simulink model "MIR_AUVSimulator_R2021b"  (R2022b)
settings: Solver=ode4  StartTime=SimuParameters.beginning_time_s  StopTime=SimuParameters.simulation_time_s  FixedStep=SimuParameters.sample_time_s  RelTol=1e-3
values from neighbouring files (symbols this model uses):
  command_parameters = loadjson('PilotParameters.json')    [Example_RunSimulation.m]    (also in RunSimulation.m)
  noise = ApplyNoise(SimuParameters.sample_time_s)    [Example_RunSimulation.m]    (also in RunSimulation.m)
  veh_model = loadjson('Conf/AUVParameters.json')    [Example_RunSimulation.m]    (also in RunSimulation.m)
undefined symbols (not defined in the file or in its folder): initial_actuators, initial_state, SimuParameters
libraries: simulink x17
settings Model: PacingRate=10  Creator=seaadh  LastModifiedBy=olanr
settings SolverCC: AlgebraicLoopSolver=TrustRegion
settings DataIOCC: ReturnWorkspaceOutputs=off
settings DebuggingCC: UnconnectedInputMsg=warning  UnconnectedOutputMsg=warning  UnconnectedLineMsg=warning  SFMachineParentedDataDiag=warning  ArithmeticOperatorsInVariantConditions=warning
settings ModelReferenceCC: UpdateModelReferenceTargets=IfOutOfDate  EnableRefExpFcnMdlSchedulingChecks=on  ModelReferenceMinAlgLoopOccurrences=on
settings SFSimCC: SimUseLocalCustomCode=off  CustomCodeUndefinedFunction=UseInterfaceOnly
settings RTWCC: RTWUseLocalCustomCode=off  DLArmComputeVersion=19.05

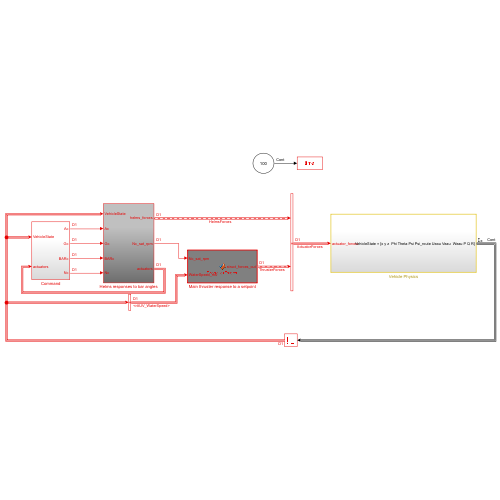
[thumbnail: Simulink's stored preview of the top-level diagram]
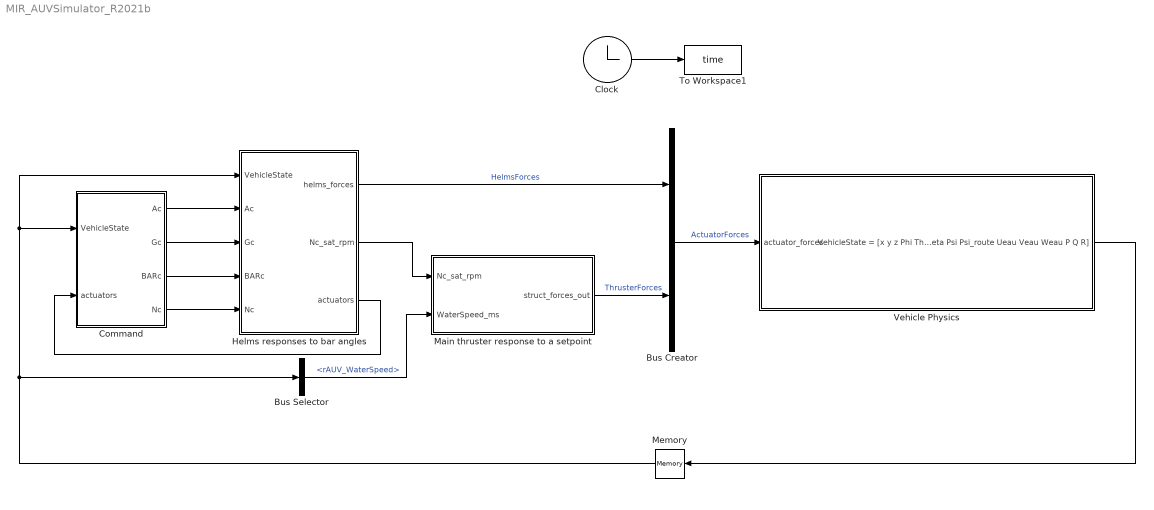
== system MIR_AUVSimulator_R2021b ==
  Bus Creator : BusCreator  Inputs=2  OutDataTypeStr=Bus: ActuatorForces
  Bus Selector : BusSelector  OutputSignals=nu.rAUV_WaterSpeed
  Clock : Clock
  Command : Subsystem
  Helms responses to bar angles : Subsystem
  Main thruster response to a setpoint : MATLAB Function  TreatAsAtomicUnit=on
  Memory : Memory  InitialCondition=initial_state  InheritSampleTime=on
  To Workspace1 : ToWorkspace  VariableName=time  SampleTime=SimuParameters.sample_time_s
  Vehicle Physics : Subsystem  TreatAsAtomicUnit=on
      settings: MinAlgLoopOccurrences=on
  wires:
  Clock/1 -> To Workspace1/1
  Memory/1 -> Helms responses to bar angles/1(VehicleState), Command/1(VehicleState), Bus Selector/1
  Helms responses to bar angles/1(helms_forces) -> Bus Creator/1  "HelmsForces"
  Helms responses to bar angles/2(Nc_sat_rpm) -> Main thruster response to a setpoint/1(Nc_sat_rpm)
  Command/1(Ac) -> Helms responses to bar angles/2(Ac)
  Command/4(Nc) -> Helms responses to bar angles/5(Nc)
  Main thruster response to a setpoint/1(struct_forces_out) -> Bus Creator/2  "ThrusterForces"
  Command/2(Gc) -> Helms responses to bar angles/3(Gc)
  Command/3(BARc) -> Helms responses to bar angles/4(BARc)
  Bus Creator/1 -> Vehicle Physics/1(actuator_forces)  "ActuatorForces"
  Vehicle Physics/1(VehicleState = [x y z Phi Theta Psi Psi_route Ueau Veau Weau P Q R]) -> Memory/1
  Bus Selector/1 -> Main thruster response to a setpoint/2(WaterSpeed_ms)  "<rAUV_WaterSpeed>"
  Helms responses to bar angles/3(actuators) -> Command/2(actuators)

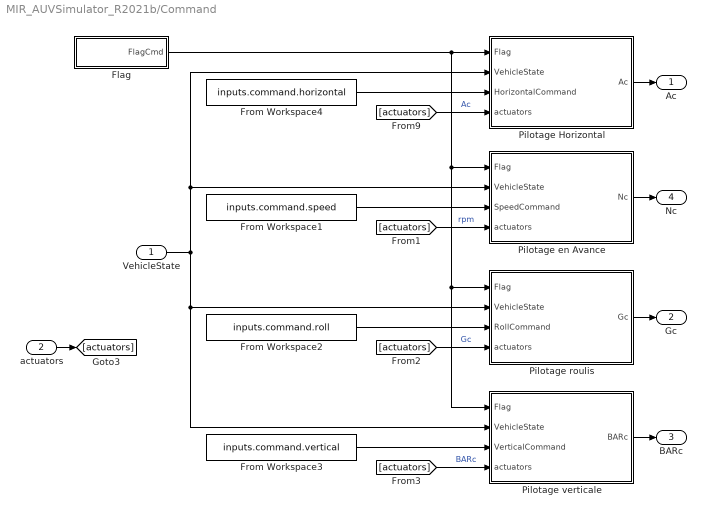
== system MIR_AUVSimulator_R2021b/Command ==
  VehicleState : Inport
  actuators : Inport  Port=2
  Flag : Subsystem
  From Workspace1 : FromWorkspace  VariableName=inputs.command.speed  SampleTime=SimuParameters.sample_time_s  Interpolate=off  OutputAfterFinalValue=Setting to zero
  From Workspace2 : FromWorkspace  VariableName=inputs.command.roll  SampleTime=SimuParameters.sample_time_s  Interpolate=off  OutputAfterFinalValue=Setting to zero
  From Workspace3 : FromWorkspace  VariableName=inputs.command.vertical  SampleTime=SimuParameters.sample_time_s  Interpolate=off  OutputAfterFinalValue=Setting to zero
  From Workspace4 : FromWorkspace  VariableName=inputs.command.horizontal  SampleTime=SimuParameters.sample_time_s  Interpolate=off  OutputAfterFinalValue=Setting to zero
  Pilotage Horizontal : Subsystem  TreatAsAtomicUnit=on  SystemSampleTime=SimuParameters.sample_time_s
  Pilotage en Avance : Subsystem  TreatAsAtomicUnit=on  SystemSampleTime=SimuParameters.sample_time_s
  Pilotage roulis : Subsystem  TreatAsAtomicUnit=on  SystemSampleTime=SimuParameters.sample_time_s
  Pilotage verticale : Subsystem  TreatAsAtomicUnit=on  SystemSampleTime=SimuParameters.sample_time_s
  Ac : Outport  VectorParamsAs1DForOutWhenUnconnected=off
  Gc : Outport  Port=2  VectorParamsAs1DForOutWhenUnconnected=off
  BARc : Outport  Port=3  VectorParamsAs1DForOutWhenUnconnected=off
  Nc : Outport  Port=4  VectorParamsAs1DForOutWhenUnconnected=off
  wires:
  Flag/1(FlagCmd) -> Pilotage verticale/1(Flag), Pilotage roulis/1(Flag), Pilotage en Avance/1(Flag), Pilotage Horizontal/1(Flag)
  Pilotage verticale/1(BARc) -> BARc/1
  Pilotage roulis/1(Gc) -> Gc/1
  Pilotage Horizontal/1(Ac) -> Ac/1
  From Workspace4/1 -> Pilotage Horizontal/3(HorizontalCommand)
  From Workspace3/1 -> Pilotage verticale/3(VerticalCommand)
  Pilotage en Avance/1(Nc) -> Nc/1
  VehicleState/1 -> Pilotage Horizontal/2(VehicleState), Pilotage en Avance/2(VehicleState), Pilotage verticale/2(VehicleState), Pilotage roulis/2(VehicleState)
  From Workspace1/1 -> Pilotage en Avance/3(SpeedCommand)
  From Workspace2/1 -> Pilotage roulis/3(RollCommand)
  actuators/1 -> [actuators]
  [actuators] -> Pilotage Horizontal/4(actuators)  "Ac"
  [actuators] -> Pilotage en Avance/4(actuators)  "rpm"
  [actuators] -> Pilotage roulis/4(actuators)  "Gc"
  [actuators] -> Pilotage verticale/4(actuators)  "BARc"

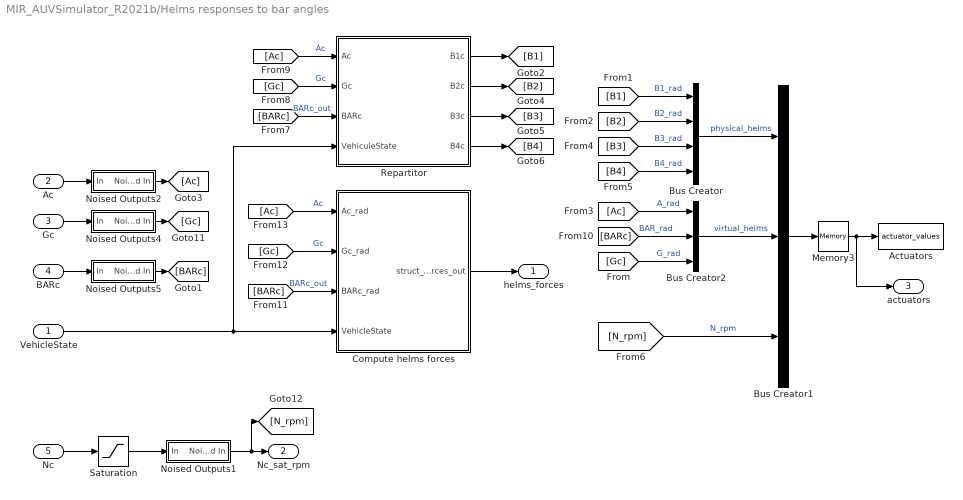
== system MIR_AUVSimulator_R2021b/Helms responses to bar angles ==
  VehicleState : Inport
  Ac : Inport  Port=2
  Gc : Inport  Port=3
  BARc : Inport  Port=4
  Nc : Inport  Port=5
  Actuators : ToWorkspace  VariableName=actuator_values  SaveFormat=Timeseries  SampleTime=SimuParameters.sample_time_s
  Bus Creator : BusCreator  Inputs=4  OutDataTypeStr=Bus: physical_helms
  Bus Creator1 : BusCreator  Inputs=3  OutDataTypeStr=Bus: ActuatorState
  Bus Creator2 : BusCreator  Inputs=3  OutDataTypeStr=Bus: virtual_helms
  Compute helms forces : MATLAB Function  TreatAsAtomicUnit=on
  Memory3 : Memory  InitialCondition=initial_actuators  InheritSampleTime=on
  Noised Outputs1 : Subsystem  mask{noise_variable=noise.RPM}
      mask prompts: noise_variable "Variable to noise"
  Noised Outputs2 : Subsystem  mask{noise_variable=noise.A_rad}
      mask prompts: noise_variable "Variable to noise"
  Noised Outputs4 : Subsystem  mask{noise_variable=noise.G_rad}
      mask prompts: noise_variable "Variable to noise"
  Noised Outputs5 : Subsystem  mask{noise_variable=noise.BAR_rad}
      mask prompts: noise_variable "Variable to noise"
  Repartitor : MATLAB Function  TreatAsAtomicUnit=on  SystemSampleTime=SimuParameters.sample_time_s
  Saturation : Saturate  UpperLimit=veh_model.Propeller.rpm_sat(2)  LowerLimit=veh_model.Propeller.rpm_sat(1)
  helms_forces : Outport  VectorParamsAs1DForOutWhenUnconnected=off
  Nc_sat_rpm : Outport  Port=2  VectorParamsAs1DForOutWhenUnconnected=off
  actuators : Outport  Port=3  VectorParamsAs1DForOutWhenUnconnected=off
  wires:
  VehicleState/1 -> Compute helms forces/4(VehicleState), Repartitor/4(VehiculeState)
  Compute helms forces/1(struct_forces_out) -> helms_forces/1
  Bus Creator1/1 -> Memory3/1
  [B3] -> Bus Creator/3  "B3_rad"
  [B2] -> Bus Creator/2  "B2_rad"
  [B4] -> Bus Creator/4  "B4_rad"
  [B1] -> Bus Creator/1  "B1_rad"
  Saturation/1 -> Noised Outputs1/1(In)
  Noised Outputs1/1(Noised In) -> [N_rpm], Nc_sat_rpm/1
  Repartitor/2(B2c) -> [B2]
  Repartitor/1(B1c) -> [B1]
  Repartitor/3(B3c) -> [B3]
  Repartitor/4(B4c) -> [B4]
  [Ac] -> Compute helms forces/1(Ac_rad)  "Ac"
  [Gc] -> Compute helms forces/2(Gc_rad)  "Gc"
  [Ac] -> Repartitor/1(Ac)  "Ac"
  [Gc] -> Repartitor/2(Gc)  "Gc"
  [BARc] -> Repartitor/3(BARc)  "BARc_out"
  [Ac] -> Bus Creator2/1  "A_rad"
  [BARc] -> Bus Creator2/2  "BAR_rad"
  [Gc] -> Bus Creator2/3  "G_rad"
  [N_rpm] -> Bus Creator1/3  "N_rpm"
  [BARc] -> Compute helms forces/3(BARc_rad)  "BARc_out"
  Bus Creator/1 -> Bus Creator1/1  "physical_helms"
  Bus Creator2/1 -> Bus Creator1/2  "virtual_helms"
  Noised Outputs2/1(Noised In) -> [Ac]
  Noised Outputs4/1(Noised In) -> [Gc]
  Noised Outputs5/1(Noised In) -> [BARc]
  Nc/1 -> Saturation/1
  Ac/1 -> Noised Outputs2/1(In)
  Gc/1 -> Noised Outputs4/1(In)
  BARc/1 -> Noised Outputs5/1(In)
  Memory3/1 -> actuators/1, Actuators/1

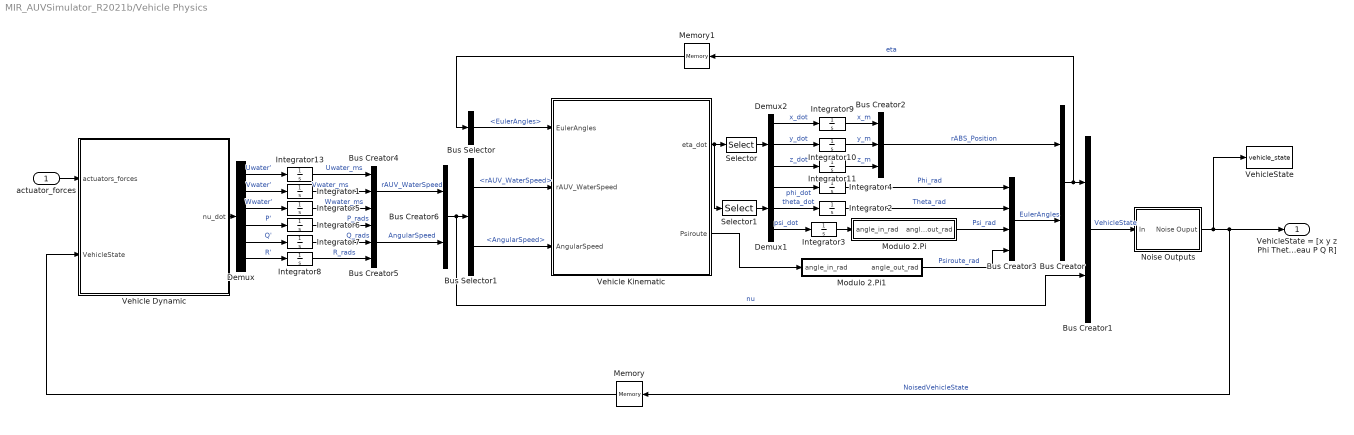
== system MIR_AUVSimulator_R2021b/Vehicle Physics ==
  actuator_forces : Inport
  Bus Creator : BusCreator  Inputs=2  OutDataTypeStr=Bus: eta
  Bus Creator1 : BusCreator  Inputs=2  OutDataTypeStr=Bus: VehicleState
  Bus Creator2 : BusCreator  Inputs=3
  Bus Creator3 : BusCreator  Inputs=4
  Bus Creator4 : BusCreator  Inputs=3
  Bus Creator5 : BusCreator  Inputs=3
  Bus Creator6 : BusCreator  Inputs=2  OutDataTypeStr=Bus: nu
  Bus Selector : BusSelector  OutputSignals=EulerAngles
  Bus Selector1 : BusSelector  OutputSignals=rAUV_WaterSpeed,AngularSpeed
  Demux : Demux  Outputs=6
  Demux1 : Demux  Outputs=3
  Demux2 : Demux  Outputs=3
  Integrator1 : Integrator  InitialCondition=initial_state.nu.rAUV_WaterSpeed.Vwater_ms  ContinuousStateAttributes='Vwater_ms'
  Integrator10 : Integrator  InitialCondition=initial_state.eta.rABS_Position.y_m  ContinuousStateAttributes='y_m'
  Integrator11 : Integrator  InitialCondition=initial_state.eta.rABS_Position.z_m  ContinuousStateAttributes='z_m'
  Integrator13 : Integrator  InitialCondition=initial_state.nu.rAUV_WaterSpeed.Uwater_ms  ContinuousStateAttributes='Uwater_ms'
  Integrator2 : Integrator  InitialCondition=initial_state.eta.EulerAngles.Theta_rad  ContinuousStateAttributes='theta_rad'
  Integrator3 : Integrator  InitialCondition=initial_state.eta.EulerAngles.Psi_rad  ContinuousStateAttributes='psi_rad'
  Integrator4 : Integrator  InitialCondition=initial_state.eta.EulerAngles.Phi_rad  ContinuousStateAttributes='phi_rad'
  Integrator5 : Integrator  InitialCondition=initial_state.nu.rAUV_WaterSpeed.Wwater_ms  ContinuousStateAttributes='Wwater_ms'
  Integrator6 : Integrator  InitialCondition=initial_state.nu.AngularSpeed.P_rads  ContinuousStateAttributes='P_rads'
  Integrator7 : Integrator  InitialCondition=initial_state.nu.AngularSpeed.Q_rads  ContinuousStateAttributes='Q_rads'
  Integrator8 : Integrator  InitialCondition=initial_state.nu.AngularSpeed.R_rads  ContinuousStateAttributes='R_rads'
  Integrator9 : Integrator  InitialCondition=initial_state.eta.rABS_Position.x_m  ContinuousStateAttributes='x_m'
  Memory : Memory  InitialCondition=initial_state  InheritSampleTime=on
  Memory1 : Memory  InitialCondition=initial_state.eta  InheritSampleTime=on
  Modulo 2.Pi : MATLAB Function  TreatAsAtomicUnit=on
  Modulo 2.Pi1 : MATLAB Function  TreatAsAtomicUnit=on
  Noise Outputs : Subsystem
  Selector : Selector  InputPortWidth=6  IndexOptions=Index vector (dialog)  Indices=[1 2 3]  OutputSizes=1
  Selector1 : Selector  InputPortWidth=6  IndexOptions=Index vector (dialog)  Indices=[4 5 6]  OutputSizes=1
  Vehicle Dynamic : Subsystem  TreatAsAtomicUnit=on
  Vehicle Kinematic : MATLAB Function  TreatAsAtomicUnit=on
  VehicleState : ToWorkspace  VariableName=vehicle_state  SaveFormat=Timeseries  SampleTime=SimuParameters.sample_time_s
  VehicleState = [x y z Phi Theta Psi Psi_route Ueau Veau Weau P Q R] : Outport  VectorParamsAs1DForOutWhenUnconnected=off
  wires:
  Demux2/1 -> Integrator9/1  "x_dot"
  Bus Creator4/1 -> Bus Creator6/1  "rAUV_WaterSpeed"
  Demux2/3 -> Integrator11/1  "z_dot"
  Bus Creator5/1 -> Bus Creator6/2  "AngularSpeed"
  Demux/6 -> Integrator8/1  "R'"
  Bus Creator6/1 -> Bus Creator1/2, Bus Selector1/1  "nu"
  Bus Selector1/1 -> Vehicle Kinematic/2(rAUV_WaterSpeed)  "<rAUV_WaterSpeed>"
  Demux/5 -> Integrator7/1  "Q'"
  Demux/2 -> Integrator1/1  "Vwater'"
  Demux/1 -> Integrator13/1  "Uwater'"
  Integrator1/1 -> Bus Creator4/2  "Vwater_ms"
  Demux/4 -> Integrator6/1  "P'"
  Bus Selector1/2 -> Vehicle Kinematic/3(AngularSpeed)  "<AngularSpeed>"
  Bus Creator2/1 -> Bus Creator/1  "rABS_Position"
  Demux2/2 -> Integrator10/1  "y_dot"
  Bus Creator/1 -> Memory1/1, Bus Creator1/1  "eta"
  Integrator5/1 -> Bus Creator4/3  "Wwater_ms"
  Bus Selector/1 -> Vehicle Kinematic/1(EulerAngles)  "<EulerAngles>"
  Bus Creator3/1 -> Bus Creator/2  "EulerAngles"
  Vehicle Dynamic/1(nu_dot) -> Demux/1
  Demux/3 -> Integrator5/1  "Wwater'"
  Bus Creator1/1 -> Noise Outputs/1(In)  "VehicleState"
  Memory/1 -> Vehicle Dynamic/2(VehicleState)
  Integrator8/1 -> Bus Creator5/3  "R_rads"
  Integrator13/1 -> Bus Creator4/1  "Uwater_ms"
  Noise Outputs/1(Noise Ouput) -> VehicleState = [x y z Phi Theta Psi Psi_route Ueau Veau Weau P Q R]/1, Memory/1, VehicleState/1  "NoisedVehicleState"
  Integrator6/1 -> Bus Creator5/1  "P_rads"
  Integrator7/1 -> Bus Creator5/2  "Q_rads"
  Memory1/1 -> Bus Selector/1
  Vehicle Kinematic/1(eta_dot) -> Selector1/1, Selector/1
  actuator_forces/1 -> Vehicle Dynamic/1(actuators_forces)
  Integrator9/1 -> Bus Creator2/1  "x_m"
  Integrator10/1 -> Bus Creator2/2  "y_m"
  Integrator11/1 -> Bus Creator2/3  "z_m"
  Selector/1 -> Demux2/1
  Demux1/3 -> Integrator3/1  "psi_dot"
  Demux1/2 -> Integrator2/1  "theta_dot"
  Demux1/1 -> Integrator4/1  "phi_dot"
  Selector1/1 -> Demux1/1
  Integrator3/1 -> Modulo 2.Pi/1(angle_in_rad)
  Modulo 2.Pi/1(angle_out_rad) -> Bus Creator3/3  "Psi_rad"
  Modulo 2.Pi1/1(angle_out_rad) -> Bus Creator3/4  "Psiroute_rad"
  Vehicle Kinematic/2(Psiroute) -> Modulo 2.Pi1/1(angle_in_rad)
  Integrator4/1 -> Bus Creator3/1  "Phi_rad"
  Integrator2/1 -> Bus Creator3/2  "Theta_rad"

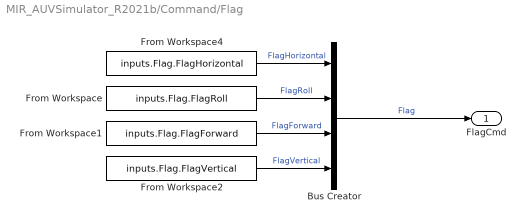
== system MIR_AUVSimulator_R2021b/Command/Flag ==
  Bus Creator : BusCreator  Inputs=4  OutDataTypeStr=Bus: Flag
  From Workspace : FromWorkspace  VariableName=inputs.Flag.FlagRoll  SampleTime=SimuParameters.sample_time_s
  From Workspace1 : FromWorkspace  VariableName=inputs.Flag.FlagForward  SampleTime=SimuParameters.sample_time_s
  From Workspace2 : FromWorkspace  VariableName=inputs.Flag.FlagVertical  SampleTime=SimuParameters.sample_time_s
  From Workspace4 : FromWorkspace  VariableName=inputs.Flag.FlagHorizontal  SampleTime=SimuParameters.sample_time_s
  FlagCmd : Outport  VectorParamsAs1DForOutWhenUnconnected=off
  wires:
  Bus Creator/1 -> FlagCmd/1  "Flag"
  From Workspace4/1 -> Bus Creator/1  "FlagHorizontal"
  From Workspace/1 -> Bus Creator/2  "FlagRoll"
  From Workspace1/1 -> Bus Creator/3  "FlagForward"
  From Workspace2/1 -> Bus Creator/4  "FlagVertical"

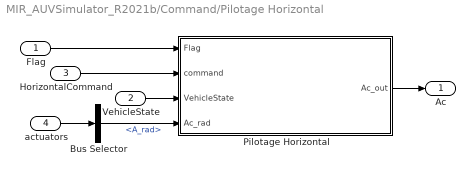
== system MIR_AUVSimulator_R2021b/Command/Pilotage Horizontal ==
  Flag : Inport
  VehicleState : Inport  Port=2
  HorizontalCommand : Inport  Port=3
  actuators : Inport  Port=4
  Bus Selector : BusSelector  OutputSignals=virtual_helms.A_rad
  Pilotage Horizontal : MATLAB Function  TreatAsAtomicUnit=on  SystemSampleTime=SimuParameters.sample_time_s
  Ac : Outport  VectorParamsAs1DForOutWhenUnconnected=off
  wires:
  Pilotage Horizontal/1(Ac_out) -> Ac/1
  HorizontalCommand/1 -> Pilotage Horizontal/2(command)
  VehicleState/1 -> Pilotage Horizontal/3(VehicleState)
  Flag/1 -> Pilotage Horizontal/1(Flag)
  actuators/1 -> Bus Selector/1
  Bus Selector/1 -> Pilotage Horizontal/4(Ac_rad)  "<A_rad>"

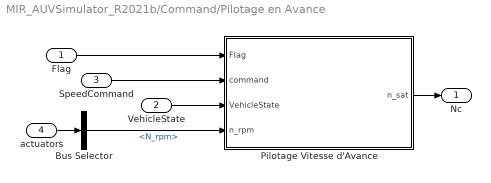
== system MIR_AUVSimulator_R2021b/Command/Pilotage en Avance ==
  Flag : Inport
  VehicleState : Inport  Port=2
  SpeedCommand : Inport  Port=3
  actuators : Inport  Port=4
  Bus Selector : BusSelector  OutputSignals=N_rpm
  Pilotage Vitesse d'Avance : MATLAB Function  TreatAsAtomicUnit=on  SystemSampleTime=SimuParameters.sample_time_s
  Nc : Outport  VectorParamsAs1DForOutWhenUnconnected=off
  wires:
  Pilotage Vitesse d'Avance/1(n_sat) -> Nc/1
  VehicleState/1 -> Pilotage Vitesse d'Avance/3(VehicleState)
  Flag/1 -> Pilotage Vitesse d'Avance/1(Flag)
  SpeedCommand/1 -> Pilotage Vitesse d'Avance/2(command)
  actuators/1 -> Bus Selector/1
  Bus Selector/1 -> Pilotage Vitesse d'Avance/4(n_rpm)  "<N_rpm>"

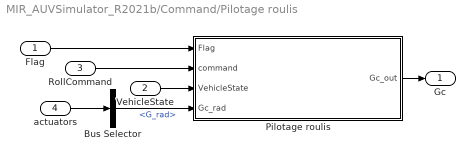
== system MIR_AUVSimulator_R2021b/Command/Pilotage roulis ==
  Flag : Inport
  VehicleState : Inport  Port=2
  RollCommand : Inport  Port=3
  actuators : Inport  Port=4
  Bus Selector : BusSelector  OutputSignals=virtual_helms.G_rad
  Pilotage roulis : MATLAB Function  TreatAsAtomicUnit=on  SystemSampleTime=SimuParameters.sample_time_s
  Gc : Outport  VectorParamsAs1DForOutWhenUnconnected=off
  wires:
  Pilotage roulis/1(Gc_out) -> Gc/1
  Flag/1 -> Pilotage roulis/1(Flag)
  VehicleState/1 -> Pilotage roulis/3(VehicleState)
  RollCommand/1 -> Pilotage roulis/2(command)
  actuators/1 -> Bus Selector/1
  Bus Selector/1 -> Pilotage roulis/4(Gc_rad)  "<G_rad>"

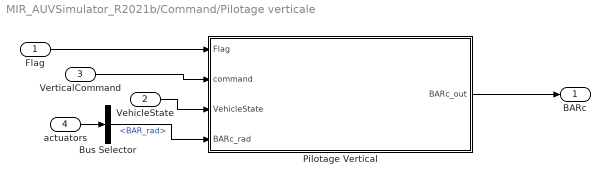
== system MIR_AUVSimulator_R2021b/Command/Pilotage verticale ==
  Flag : Inport
  VehicleState : Inport  Port=2
  VerticalCommand : Inport  Port=3
  actuators : Inport  Port=4
  Bus Selector : BusSelector  OutputSignals=virtual_helms.BAR_rad
  Pilotage Vertical : MATLAB Function  TreatAsAtomicUnit=on  SystemSampleTime=SimuParameters.sample_time_s
  BARc : Outport  VectorParamsAs1DForOutWhenUnconnected=off
  wires:
  Pilotage Vertical/1(BARc_out) -> BARc/1
  Flag/1 -> Pilotage Vertical/1(Flag)
  VehicleState/1 -> Pilotage Vertical/3(VehicleState)
  VerticalCommand/1 -> Pilotage Vertical/2(command)
  actuators/1 -> Bus Selector/1
  Bus Selector/1 -> Pilotage Vertical/4(BARc_rad)  "<BAR_rad>"

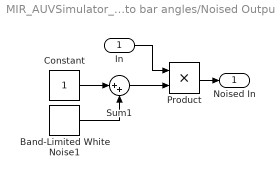
== system MIR_AUVSimulator_R2021b/Helms responses to bar angles/Noised Outputs1 ==
  In : Inport
  Band-Limited White Noise1 : simulink/Sources/Band-Limited White Noise  Cov=noise_variable.noise_power  Ts=SimuParameters.sample_time_s  seed=[23341]
  Constant : Constant
  Product : Product
  Sum1 : Sum  Inputs=|++
  Noised In : Outport  VectorParamsAs1DForOutWhenUnconnected=off
  wires:
  Product/1 -> Noised In/1
  In/1 -> Product/1
  Constant/1 -> Sum1/1
  Band-Limited White Noise1/1 -> Sum1/2
  Sum1/1 -> Product/2

== system MIR_AUVSimulator_R2021b/Helms responses to bar angles/Noised Outputs2 ==
  In : Inport
  Band-Limited White Noise1 : simulink/Sources/Band-Limited White Noise  Cov=noise_variable.noise_power  Ts=SimuParameters.sample_time_s  seed=[23341]
  Constant : Constant
  Product : Product
  Sum1 : Sum  Inputs=|++
  Noised In : Outport  VectorParamsAs1DForOutWhenUnconnected=off
  wires:
  Product/1 -> Noised In/1
  In/1 -> Product/1
  Constant/1 -> Sum1/1
  Band-Limited White Noise1/1 -> Sum1/2
  Sum1/1 -> Product/2

== system MIR_AUVSimulator_R2021b/Helms responses to bar angles/Noised Outputs4 ==
  In : Inport
  Band-Limited White Noise1 : simulink/Sources/Band-Limited White Noise  Cov=noise_variable.noise_power  Ts=SimuParameters.sample_time_s  seed=[23341]
  Constant : Constant
  Product : Product
  Sum1 : Sum  Inputs=|++
  Noised In : Outport  VectorParamsAs1DForOutWhenUnconnected=off
  wires:
  Product/1 -> Noised In/1
  In/1 -> Product/1
  Constant/1 -> Sum1/1
  Band-Limited White Noise1/1 -> Sum1/2
  Sum1/1 -> Product/2

== system MIR_AUVSimulator_R2021b/Helms responses to bar angles/Noised Outputs5 ==
  In : Inport
  Band-Limited White Noise1 : simulink/Sources/Band-Limited White Noise  Cov=noise_variable.noise_power  Ts=SimuParameters.sample_time_s  seed=[23341]
  Constant : Constant
  Product : Product
  Sum1 : Sum  Inputs=|++
  Noised In : Outport  VectorParamsAs1DForOutWhenUnconnected=off
  wires:
  Product/1 -> Noised In/1
  In/1 -> Product/1
  Constant/1 -> Sum1/1
  Band-Limited White Noise1/1 -> Sum1/2
  Sum1/1 -> Product/2

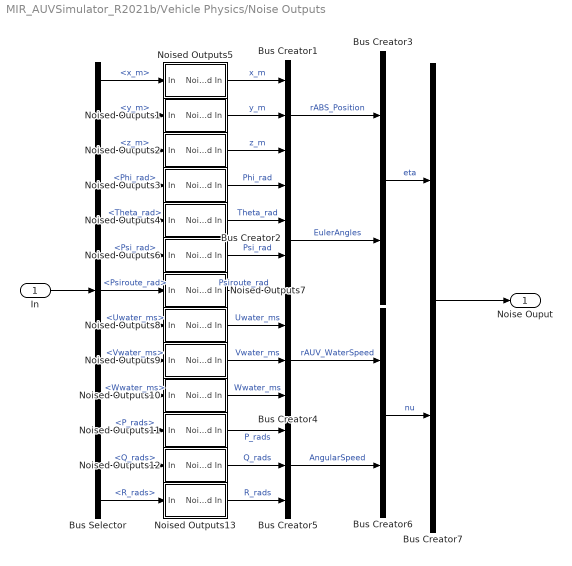
== system MIR_AUVSimulator_R2021b/Vehicle Physics/Noise Outputs ==
  In : Inport
  Bus Creator1 : BusCreator  Inputs=3  OutDataTypeStr=Bus: rABS_Position
  Bus Creator2 : BusCreator  Inputs=4  OutDataTypeStr=Bus: EulerAngles
  Bus Creator3 : BusCreator  Inputs=2  OutDataTypeStr=Bus: eta
  Bus Creator4 : BusCreator  Inputs=3  OutDataTypeStr=Bus: rAUV_WaterSpeed
  Bus Creator5 : BusCreator  Inputs=3  OutDataTypeStr=Bus: AngularSpeed
  Bus Creator6 : BusCreator  Inputs=2  OutDataTypeStr=Bus: nu
  Bus Creator7 : BusCreator  Inputs=2  OutDataTypeStr=Bus: VehicleState
  Bus Selector : BusSelector  OutputSignals=eta.rABS_Position.x_m,eta.rABS_Position.y_m,eta.rABS_Position.z_m,eta.EulerAngles.Phi_rad,eta.EulerAngles.Theta_rad,eta.EulerAngles.Psi_rad,eta.EulerAngles.Psiroute_rad,nu.rAUV_WaterSpeed.Uwater_ms,nu.rAUV_WaterSpeed.Vwater_ms,nu.rAUV_WaterSpeed.Wwater_ms,nu.AngularSpeed.P_rads,nu.AngularSpeed.Q_rads,nu.AngularSpeed.R_rads
  Noised Outputs1 : Subsystem  mask{noise_variable=noise.y_m}
      mask prompts: noise_variable "Variable to noise"
  Noised Outputs10 : Subsystem  mask{noise_variable=noise.Weau_ms}
      mask prompts: noise_variable "Variable to noise"
  Noised Outputs11 : Subsystem  mask{noise_variable=noise.P_rads}
      mask prompts: noise_variable "Variable to noise"
  Noised Outputs12 : Subsystem  mask{noise_variable=noise.Q_rads}
      mask prompts: noise_variable "Variable to noise"
  Noised Outputs13 : Subsystem  mask{noise_variable=noise.R_rads}
      mask prompts: noise_variable "Variable to noise"
  Noised Outputs2 : Subsystem  mask{noise_variable=noise.z_m}
      mask prompts: noise_variable "Variable to noise"
  Noised Outputs3 : Subsystem  mask{noise_variable=noise.Phi_rad}
      mask prompts: noise_variable "Variable to noise"
  Noised Outputs4 : Subsystem  mask{noise_variable=noise.Theta_rad}
      mask prompts: noise_variable "Variable to noise"
  Noised Outputs5 : Subsystem  mask{noise_variable=noise.x_m}
      mask prompts: noise_variable "Variable to noise"
  Noised Outputs6 : Subsystem  mask{noise_variable=noise.Psi_rad}
      mask prompts: noise_variable "Variable to noise"
  Noised Outputs7 : Subsystem  mask{noise_variable=noise.Psiroute_rad}
      mask prompts: noise_variable "Variable to noise"
  Noised Outputs8 : Subsystem  mask{noise_variable=noise.Ueau_ms}
      mask prompts: noise_variable "Variable to noise"
  Noised Outputs9 : Subsystem  mask{noise_variable=noise.Veau_ms}
      mask prompts: noise_variable "Variable to noise"
  Noise Ouput : Outport  VectorParamsAs1DForOutWhenUnconnected=off
  wires:
  Noised Outputs9/1(Noised In) -> Bus Creator4/2  "Vwater_ms"
  Noised Outputs8/1(Noised In) -> Bus Creator4/1  "Uwater_ms"
  Noised Outputs10/1(Noised In) -> Bus Creator4/3  "Wwater_ms"
  Bus Creator5/1 -> Bus Creator6/2  "AngularSpeed"
  Bus Creator4/1 -> Bus Creator6/1  "rAUV_WaterSpeed"
  Noised Outputs11/1(Noised In) -> Bus Creator5/1  "P_rads"
  Noised Outputs12/1(Noised In) -> Bus Creator5/2  "Q_rads"
  Noised Outputs13/1(Noised In) -> Bus Creator5/3  "R_rads"
  Bus Creator3/1 -> Bus Creator7/1  "eta"
  Bus Creator2/1 -> Bus Creator3/2  "EulerAngles"
  Noised Outputs5/1(Noised In) -> Bus Creator1/1  "x_m"
  Bus Creator1/1 -> Bus Creator3/1  "rABS_Position"
  Noised Outputs1/1(Noised In) -> Bus Creator1/2  "y_m"
  Noised Outputs2/1(Noised In) -> Bus Creator1/3  "z_m"
  Noised Outputs3/1(Noised In) -> Bus Creator2/1  "Phi_rad"
  Noised Outputs6/1(Noised In) -> Bus Creator2/3  "Psi_rad"
  Noised Outputs4/1(Noised In) -> Bus Creator2/2  "Theta_rad"
  In/1 -> Bus Selector/1
  Bus Creator7/1 -> Noise Ouput/1
  Bus Selector/1 -> Noised Outputs5/1(In)  "<x_m>"
  Bus Selector/2 -> Noised Outputs1/1(In)  "<y_m>"
  Bus Selector/3 -> Noised Outputs2/1(In)  "<z_m>"
  Bus Selector/4 -> Noised Outputs3/1(In)  "<Phi_rad>"
  Bus Selector/5 -> Noised Outputs4/1(In)  "<Theta_rad>"
  Bus Selector/6 -> Noised Outputs6/1(In)  "<Psi_rad>"
  Bus Selector/7 -> Noised Outputs7/1(In)  "<Psiroute_rad>"
  Noised Outputs7/1(Noised In) -> Bus Creator2/4  "Psiroute_rad"
  Bus Creator6/1 -> Bus Creator7/2  "nu"
  Bus Selector/8 -> Noised Outputs8/1(In)  "<Uwater_ms>"
  Bus Selector/9 -> Noised Outputs9/1(In)  "<Vwater_ms>"
  Bus Selector/10 -> Noised Outputs10/1(In)  "<Wwater_ms>"
  Bus Selector/11 -> Noised Outputs11/1(In)  "<P_rads>"
  Bus Selector/12 -> Noised Outputs12/1(In)  "<Q_rads>"
  Bus Selector/13 -> Noised Outputs13/1(In)  "<R_rads>"

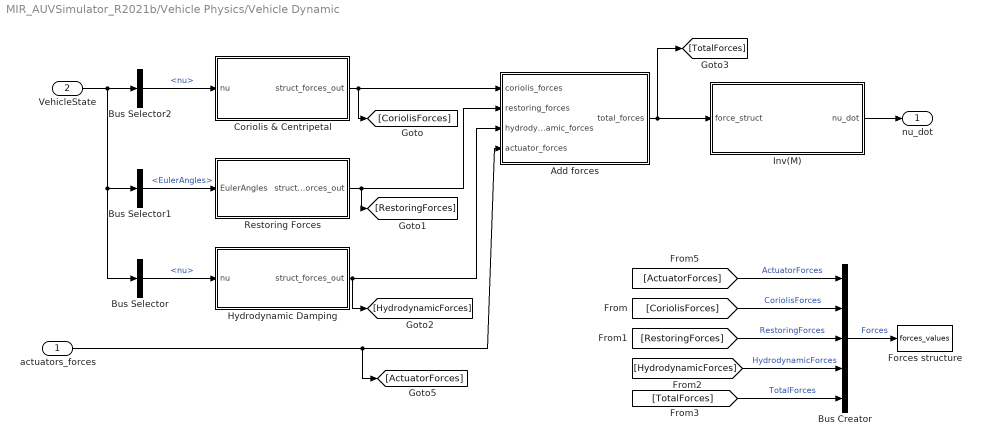
== system MIR_AUVSimulator_R2021b/Vehicle Physics/Vehicle Dynamic ==
  actuators_forces : Inport
  VehicleState : Inport  Port=2
  Add forces : MATLAB Function  TreatAsAtomicUnit=on
  Bus Creator : BusCreator  Inputs=5  OutDataTypeStr=Bus: Forces
  Bus Selector : BusSelector  OutputSignals=nu
  Bus Selector1 : BusSelector  OutputSignals=eta.EulerAngles
  Bus Selector2 : BusSelector  OutputSignals=nu
  Coriolis & Centripetal : MATLAB Function  TreatAsAtomicUnit=on
  Forces structure : ToWorkspace  VariableName=forces_values  SaveFormat=Timeseries  SampleTime=SimuParameters.sample_time_s
  Hydrodynamic Damping : MATLAB Function  TreatAsAtomicUnit=on
  Inv(M) : MATLAB Function  TreatAsAtomicUnit=on
  Restoring Forces : MATLAB Function  TreatAsAtomicUnit=on
  nu_dot : Outport  VectorParamsAs1DForOutWhenUnconnected=off
  wires:
  VehicleState/1 -> Bus Selector2/1, Bus Selector/1, Bus Selector1/1
  Inv(M)/1(nu_dot) -> nu_dot/1
  Bus Selector/1 -> Hydrodynamic Damping/1(nu)  "<nu>"
  Bus Selector2/1 -> Coriolis & Centripetal/1(nu)  "<nu>"
  Bus Selector1/1 -> Restoring Forces/1(EulerAngles)  "<EulerAngles>"
  Coriolis & Centripetal/1(struct_forces_out) -> [CoriolisForces], Add forces/1(coriolis_forces)
  Restoring Forces/1(struct_forces_out) -> Add forces/2(restoring_forces), [RestoringForces]
  Hydrodynamic Damping/1(struct_forces_out) -> [HydrodynamicForces], Add forces/3(hydrodynamic_forces)
  [ActuatorForces] -> Bus Creator/1  "ActuatorForces"
  [CoriolisForces] -> Bus Creator/2  "CoriolisForces"
  [RestoringForces] -> Bus Creator/3  "RestoringForces"
  Bus Creator/1 -> Forces structure/1  "Forces"
  actuators_forces/1 -> Add forces/4(actuator_forces), [ActuatorForces]
  [HydrodynamicForces] -> Bus Creator/4  "HydrodynamicForces"
  [TotalForces] -> Bus Creator/5  "TotalForces"
  Add forces/1(total_forces) -> Inv(M)/1(force_struct), [TotalForces]

== system MIR_AUVSimulator_R2021b/Vehicle Physics/Noise Outputs/Noised Outputs1 ==
  In : Inport
  Band-Limited White Noise1 : simulink/Sources/Band-Limited White Noise  Cov=noise_variable.noise_power  Ts=SimuParameters.sample_time_s  seed=[23341]
  Constant : Constant
  Product : Product
  Sum1 : Sum  Inputs=|++
  Noised In : Outport  VectorParamsAs1DForOutWhenUnconnected=off
  wires:
  Product/1 -> Noised In/1
  In/1 -> Product/1
  Constant/1 -> Sum1/1
  Band-Limited White Noise1/1 -> Sum1/2
  Sum1/1 -> Product/2

== system MIR_AUVSimulator_R2021b/Vehicle Physics/Noise Outputs/Noised Outputs10 ==
  In : Inport
  Band-Limited White Noise1 : simulink/Sources/Band-Limited White Noise  Cov=noise_variable.noise_power  Ts=SimuParameters.sample_time_s  seed=[23341]
  Constant : Constant
  Product : Product
  Sum1 : Sum  Inputs=|++
  Noised In : Outport  VectorParamsAs1DForOutWhenUnconnected=off
  wires:
  Product/1 -> Noised In/1
  In/1 -> Product/1
  Constant/1 -> Sum1/1
  Band-Limited White Noise1/1 -> Sum1/2
  Sum1/1 -> Product/2

== system MIR_AUVSimulator_R2021b/Vehicle Physics/Noise Outputs/Noised Outputs11 ==
  In : Inport
  Band-Limited White Noise1 : simulink/Sources/Band-Limited White Noise  Cov=noise_variable.noise_power  Ts=SimuParameters.sample_time_s  seed=[23341]
  Constant : Constant
  Product : Product
  Sum1 : Sum  Inputs=|++
  Noised In : Outport  VectorParamsAs1DForOutWhenUnconnected=off
  wires:
  Product/1 -> Noised In/1
  In/1 -> Product/1
  Constant/1 -> Sum1/1
  Band-Limited White Noise1/1 -> Sum1/2
  Sum1/1 -> Product/2

== system MIR_AUVSimulator_R2021b/Vehicle Physics/Noise Outputs/Noised Outputs12 ==
  In : Inport
  Band-Limited White Noise1 : simulink/Sources/Band-Limited White Noise  Cov=noise_variable.noise_power  Ts=SimuParameters.sample_time_s  seed=[23341]
  Constant : Constant
  Product : Product
  Sum1 : Sum  Inputs=|++
  Noised In : Outport  VectorParamsAs1DForOutWhenUnconnected=off
  wires:
  Product/1 -> Noised In/1
  In/1 -> Product/1
  Constant/1 -> Sum1/1
  Band-Limited White Noise1/1 -> Sum1/2
  Sum1/1 -> Product/2

== system MIR_AUVSimulator_R2021b/Vehicle Physics/Noise Outputs/Noised Outputs13 ==
  In : Inport
  Band-Limited White Noise1 : simulink/Sources/Band-Limited White Noise  Cov=noise_variable.noise_power  Ts=SimuParameters.sample_time_s  seed=[23341]
  Constant : Constant
  Product : Product
  Sum1 : Sum  Inputs=|++
  Noised In : Outport  VectorParamsAs1DForOutWhenUnconnected=off
  wires:
  Product/1 -> Noised In/1
  In/1 -> Product/1
  Constant/1 -> Sum1/1
  Band-Limited White Noise1/1 -> Sum1/2
  Sum1/1 -> Product/2

== system MIR_AUVSimulator_R2021b/Vehicle Physics/Noise Outputs/Noised Outputs2 ==
  In : Inport
  Band-Limited White Noise1 : simulink/Sources/Band-Limited White Noise  Cov=noise_variable.noise_power  Ts=SimuParameters.sample_time_s  seed=[23341]
  Constant : Constant
  Product : Product
  Sum1 : Sum  Inputs=|++
  Noised In : Outport  VectorParamsAs1DForOutWhenUnconnected=off
  wires:
  Product/1 -> Noised In/1
  In/1 -> Product/1
  Constant/1 -> Sum1/1
  Band-Limited White Noise1/1 -> Sum1/2
  Sum1/1 -> Product/2

== system MIR_AUVSimulator_R2021b/Vehicle Physics/Noise Outputs/Noised Outputs3 ==
  In : Inport
  Band-Limited White Noise1 : simulink/Sources/Band-Limited White Noise  Cov=noise_variable.noise_power  Ts=SimuParameters.sample_time_s  seed=[23341]
  Constant : Constant
  Product : Product
  Sum1 : Sum  Inputs=|++
  Noised In : Outport  VectorParamsAs1DForOutWhenUnconnected=off
  wires:
  Product/1 -> Noised In/1
  In/1 -> Product/1
  Constant/1 -> Sum1/1
  Band-Limited White Noise1/1 -> Sum1/2
  Sum1/1 -> Product/2

== system MIR_AUVSimulator_R2021b/Vehicle Physics/Noise Outputs/Noised Outputs4 ==
  In : Inport
  Band-Limited White Noise1 : simulink/Sources/Band-Limited White Noise  Cov=noise_variable.noise_power  Ts=SimuParameters.sample_time_s  seed=[23341]
  Constant : Constant
  Product : Product
  Sum1 : Sum  Inputs=|++
  Noised In : Outport  VectorParamsAs1DForOutWhenUnconnected=off
  wires:
  Product/1 -> Noised In/1
  In/1 -> Product/1
  Constant/1 -> Sum1/1
  Band-Limited White Noise1/1 -> Sum1/2
  Sum1/1 -> Product/2

== system MIR_AUVSimulator_R2021b/Vehicle Physics/Noise Outputs/Noised Outputs5 ==
  In : Inport
  Band-Limited White Noise1 : simulink/Sources/Band-Limited White Noise  Cov=noise_variable.noise_power  Ts=SimuParameters.sample_time_s  seed=[23341]
  Constant : Constant
  Product : Product
  Sum1 : Sum  Inputs=|++
  Noised In : Outport  VectorParamsAs1DForOutWhenUnconnected=off
  wires:
  Product/1 -> Noised In/1
  In/1 -> Product/1
  Constant/1 -> Sum1/1
  Band-Limited White Noise1/1 -> Sum1/2
  Sum1/1 -> Product/2

== system MIR_AUVSimulator_R2021b/Vehicle Physics/Noise Outputs/Noised Outputs6 ==
  In : Inport
  Band-Limited White Noise1 : simulink/Sources/Band-Limited White Noise  Cov=noise_variable.noise_power  Ts=SimuParameters.sample_time_s  seed=[23341]
  Constant : Constant
  Product : Product
  Sum1 : Sum  Inputs=|++
  Noised In : Outport  VectorParamsAs1DForOutWhenUnconnected=off
  wires:
  Product/1 -> Noised In/1
  In/1 -> Product/1
  Constant/1 -> Sum1/1
  Band-Limited White Noise1/1 -> Sum1/2
  Sum1/1 -> Product/2

== system MIR_AUVSimulator_R2021b/Vehicle Physics/Noise Outputs/Noised Outputs7 ==
  In : Inport
  Band-Limited White Noise1 : simulink/Sources/Band-Limited White Noise  Cov=noise_variable.noise_power  Ts=SimuParameters.sample_time_s  seed=[23341]
  Constant : Constant
  Product : Product
  Sum1 : Sum  Inputs=|++
  Noised In : Outport  VectorParamsAs1DForOutWhenUnconnected=off
  wires:
  Product/1 -> Noised In/1
  In/1 -> Product/1
  Constant/1 -> Sum1/1
  Band-Limited White Noise1/1 -> Sum1/2
  Sum1/1 -> Product/2

== system MIR_AUVSimulator_R2021b/Vehicle Physics/Noise Outputs/Noised Outputs8 ==
  In : Inport
  Band-Limited White Noise1 : simulink/Sources/Band-Limited White Noise  Cov=noise_variable.noise_power  Ts=SimuParameters.sample_time_s  seed=[23341]
  Constant : Constant
  Product : Product
  Sum1 : Sum  Inputs=|++
  Noised In : Outport  VectorParamsAs1DForOutWhenUnconnected=off
  wires:
  Product/1 -> Noised In/1
  In/1 -> Product/1
  Constant/1 -> Sum1/1
  Band-Limited White Noise1/1 -> Sum1/2
  Sum1/1 -> Product/2

== system MIR_AUVSimulator_R2021b/Vehicle Physics/Noise Outputs/Noised Outputs9 ==
  In : Inport
  Band-Limited White Noise1 : simulink/Sources/Band-Limited White Noise  Cov=noise_variable.noise_power  Ts=SimuParameters.sample_time_s  seed=[23341]
  Constant : Constant
  Product : Product
  Sum1 : Sum  Inputs=|++
  Noised In : Outport  VectorParamsAs1DForOutWhenUnconnected=off
  wires:
  Product/1 -> Noised In/1
  In/1 -> Product/1
  Constant/1 -> Sum1/1
  Band-Limited White Noise1/1 -> Sum1/2
  Sum1/1 -> Product/2

== matlab function MIR_AUVSimulator_R2021b/Command/Pilotage en Avance/Pilotage Vitesse d'Avance ==
  data: Flag input; command input; VehicleState input; n_rpm input; n_sat output; SimuParameters parameter; command_parameters parameter
function n_sat = ForwardControl(Flag,command,VehicleState,n_rpm,SimuParameters,command_parameters)

persistent init memory;

speed_flag = GetFlagName(Flag.FlagForward);

%% Load inputs
in.u_ms = VehicleState.nu.rAUV_WaterSpeed.Uwater_ms;
in.uc_ms = command;
in.delta_time_s = SimuParameters.sample_time_s;

%% Memory management
if isempty(init)
    init = false;
    memory = InitPilotForwardSpeed();
end
if init
    init = false;
    memory = InitPilotForwardSpeed();
end

%% Piloting
switch speed_flag
    case 'OpenLoop'
        n_rpm = command;
        init = true;
        
    case 'ForwardSpeed'
        memory = UpdatePilotForwardSpeedMemory(in,memory,command_parameters.ForwardSpeed);
        
        out = PilotForwardSpeed(in,memory,command_parameters.ForwardSpeed);
        n_rpm = out.Nc_rpm;
end

n_sat = n_rpm;
end
function forward_speed_flag = GetFlagName(flag)
% Get the forward_speed_flag string depending on flag numeric input
forward_speed_flag = '';

switch flag
    case 0
        forward_speed_flag = 'OpenLoop';
    case 1
        forward_speed_flag = 'ForwardSpeed';   
end
end

== matlab function MIR_AUVSimulator_R2021b/Helms responses to bar angles/Compute helms forces ==
  data: Ac_rad input; Gc_rad input; BARc_rad input; VehicleState input; struct_forces_out output Bus: HelmsForces; veh_model parameter
function struct_forces_out = HelmsForces(Ac_rad,Gc_rad,BARc_rad,VehicleState,veh_model)
% Be careful. Output need to be a struct (because bus) not an array

u_ms = VehicleState.nu.rAUV_WaterSpeed.Uwater_ms;
v_ms = VehicleState.nu.rAUV_WaterSpeed.Vwater_ms;
w_ms = VehicleState.nu.rAUV_WaterSpeed.Wwater_ms;

speed_ms = [u_ms;v_ms;w_ms]; %m/s
virtual_helms = [Ac_rad;Gc_rad;BARc_rad];

%% Compute the force created by the helms
helm_param = veh_model.XRearHelms;
helm_param.Rho = veh_model.Environment.Rho;
helm_param.Sref = veh_model.Mecanic.surface_reference;
helm_param.Lref = veh_model.Mecanic.length_reference;

helms_forces = ComputeHelmsForce(helm_param, virtual_helms, speed_ms);
            
% Construct the struct output
struct_forces_out.Fx_N = helms_forces(1);
struct_forces_out.Fy_N = helms_forces(2);
struct_forces_out.Fz_N = helms_forces(3);
struct_forces_out.Mx_Nm = helms_forces(4);
struct_forces_out.My_Nm = helms_forces(5);
struct_forces_out.Mz_Nm = helms_forces(6);
end

== matlab function MIR_AUVSimulator_R2021b/Command/Pilotage verticale/Pilotage Vertical ==
  data: Flag input; command input; VehicleState input; BARc_rad input; BARc_out output; command_parameters parameter; SimuParameters parameter; veh_model parameter
function BARc_out  = VerticalControl(Flag,command,VehicleState,BARc_rad,command_parameters,SimuParameters, veh_model)

persistent init memory;

vertical_flag = GetFlagName(Flag.FlagVertical);

%% Load inputs
in.u_ms = VehicleState.nu.rAUV_WaterSpeed.Uwater_ms;
in.w_ms = VehicleState.nu.rAUV_WaterSpeed.Wwater_ms;
in.q_rads = VehicleState.nu.AngularSpeed.Q_rads;
in.theta_rad = VehicleState.eta.EulerAngles.Theta_rad;
in.z_m = VehicleState.eta.rABS_Position.z_m;
in.thetac_rad = 0.0;
in.zc_m = 0.0;
in.delta_time_s = SimuParameters.sample_time_s;

%% Memory management
if isempty(init)
    init = true;
    BARc_rad = 0;
    memory = InitPilotDepth();
end
if init
    init = false;
    memory = InitPilotDepth();
end

%% Piloting
switch vertical_flag
    case 'OpenLoop'
        BARc_rad = command;
        init = true;
        
    case 'Depth'
        in.zc_m = command;
        depth_param = command_parameters.Vertical.Depth;
        
        memory = UpdatePilotDepthMemory(in,memory,depth_param);
        
        out = PilotDepth_LQR(in,memory, depth_param, veh_model);
        BARc_rad = out.BARc;
        
    case 'Pitch'
        in.thetac_rad = command;
        
        out = PilotPitch(in, command_parameters.Vertical.Pitch);
        BARc_rad = out.BARc;
        init = true;
end

BARc_out = BARc_rad;
end


function vertical_flag = GetFlagName(flag)
% Get the vertical_flag string depending on flag numeric input
vertical_flag = '';

switch flag
    case 0
        vertical_flag = 'OpenLoop';
    case 1
        vertical_flag = 'Depth';
    case 2
        vertical_flag = 'Pitch';
end
end

== matlab function MIR_AUVSimulator_R2021b/Vehicle Physics/Vehicle Dynamic/Inv(M) ==
  data: force_struct input; nu_dot output; veh_model parameter
function nu_dot = fcn(force_struct,veh_model)

forces_vector = [...
    force_struct.Fx_N; force_struct.Fy_N; force_struct.Fz_N; ...
    force_struct.Mx_Nm; force_struct.My_Nm; force_struct.Mz_Nm];

inverse_veh_mass_matrix = GetInverseVehicleMassMatrix(veh_model.Mecanic);
nu_dot = inverse_veh_mass_matrix*forces_vector ;
end

== matlab function MIR_AUVSimulator_R2021b/Vehicle Physics/Vehicle Kinematic ==
  data: eta_dot output; EulerAngles input; rAUV_WaterSpeed input; AngularSpeed input; Psiroute output
function [eta_dot, Psiroute] = fcn(EulerAngles,rAUV_WaterSpeed,AngularSpeed)

%% Load inputs and variables
% Remember : EulerAngles = [phi theta psi]' = eta(4:6)
phi_rad = EulerAngles.Phi_rad;
theta_rad = EulerAngles.Theta_rad;
psi_rad = EulerAngles.Psi_rad;

% Remember : nu = [U V W P Q R]' = StateVector(7:12)
waterSpeed_RAUV_ms = [  rAUV_WaterSpeed.Uwater_ms;...
    rAUV_WaterSpeed.Vwater_ms;...
    rAUV_WaterSpeed.Wwater_ms];
angularSpeed_RAUV_rads = [  AngularSpeed.P_rads;...
    AngularSpeed.Q_rads;...
    AngularSpeed.R_rads];

%% Euler angle representation
nu = [waterSpeed_RAUV_ms;angularSpeed_RAUV_rads];

% Calculation of kinematic equations (Fossen 2.38), in radian
J = eulerang(phi_rad,theta_rad,psi_rad);
eta_dot = J*nu;

%% We had the COG (course over ground)
Psiroute = atan2(eta_dot(2),eta_dot(1));
end

== matlab function MIR_AUVSimulator_R2021b/Vehicle Physics/Vehicle Dynamic/Coriolis & Centripetal ==
  data: nu input; struct_forces_out output Bus: CoriolisForces; veh_model parameter

function struct_forces_out = FCoriolis(nu,veh_model)
% Be careful. output need to be a struct (because bus) not an array

%% Get speeds
speed_ms =  [  nu.rAUV_WaterSpeed.Uwater_ms;
    nu.rAUV_WaterSpeed.Vwater_ms;
    nu.rAUV_WaterSpeed.Wwater_ms;];

angular_speed_rads = [nu.AngularSpeed.P_rads;
    nu.AngularSpeed.Q_rads;
    nu.AngularSpeed.R_rads];

%% Compute forces
center_of_gravity_veh_ref = veh_model.Mecanic.center_of_gravity_veh_ref;
mass_kg =  veh_model.Mecanic.mass;
inertia_matrix =  veh_model.Mecanic.inertia_matrix;

coriolis_forces = ComputeCoriolisForces(speed_ms,angular_speed_rads, ...
    center_of_gravity_veh_ref, mass_kg,inertia_matrix);

% Construct the struct output
struct_forces_out.Fx_N = coriolis_forces(1);
struct_forces_out.Fy_N = coriolis_forces(2);
struct_forces_out.Fz_N = coriolis_forces(3);
struct_forces_out.Mx_Nm = coriolis_forces(4);
struct_forces_out.My_Nm = coriolis_forces(5);
struct_forces_out.Mz_Nm = coriolis_forces(6);

end

== matlab function MIR_AUVSimulator_R2021b/Vehicle Physics/Vehicle Dynamic/Hydrodynamic Damping ==
  data: nu input; struct_forces_out output Bus: HydrodynamicForces; veh_model parameter
function struct_forces_out = fcn(nu,veh_model)
% Be careful. output need to be a struct (because bus) not an array

%% Definition of velocity (speed and angular speed) vectors
% Remember nu=[Ueau Veau Weau P Q R]'
Uwater_ms = nu.rAUV_WaterSpeed.Uwater_ms;
Vwater_ms = nu.rAUV_WaterSpeed.Vwater_ms;
Wwater_ms = nu.rAUV_WaterSpeed.Wwater_ms;
P_rads = nu.AngularSpeed.P_rads;
Q_rads = nu.AngularSpeed.Q_rads;
R_rads = nu.AngularSpeed.R_rads;

speed_ms = [Uwater_ms; Vwater_ms; Wwater_ms];
angular_speed_rads = [P_rads; Q_rads; R_rads];

%% Create parameters
parameters = veh_model.Hydrodynamic;
parameters.Lref = veh_model.Mecanic.length_reference;
parameters.Sref = veh_model.Mecanic.surface_reference;
parameters.Rho = veh_model.Environment.Rho;
parameters.nu = veh_model.Environment.nu;

%% Compute Hydrodynamic damping forces
hydrodynamic_forces = ComputeHydrodynamicForce(speed_ms,angular_speed_rads,parameters);

% Construct the struct output
struct_forces_out.Fx_N = hydrodynamic_forces(1);
struct_forces_out.Fy_N = hydrodynamic_forces(2);
struct_forces_out.Fz_N = hydrodynamic_forces(3);
struct_forces_out.Mx_Nm = hydrodynamic_forces(4);
struct_forces_out.My_Nm = hydrodynamic_forces(5);
struct_forces_out.Mz_Nm = hydrodynamic_forces(6);
end

== matlab function MIR_AUVSimulator_R2021b/Vehicle Physics/Vehicle Dynamic/Restoring Forces ==
  data: EulerAngles input; struct_forces_out output Bus: RestoringForces; veh_model parameter
function struct_forces_out  = fcn(EulerAngles,veh_model)
% Be careful. output need to be a struct (because bus) not an array

% Simplified expression of the vector of hydrostatic forces and moments (Fossen 3.120)
restoring_forces = ComputeRestoringForce(EulerAngles,veh_model);

% Construct the struct output
struct_forces_out.Fx_N = restoring_forces(1);
struct_forces_out.Fy_N = restoring_forces(2);
struct_forces_out.Fz_N = restoring_forces(3);
struct_forces_out.Mx_Nm = restoring_forces(4);
struct_forces_out.My_Nm = restoring_forces(5);
struct_forces_out.Mz_Nm = restoring_forces(6);

end

== matlab function MIR_AUVSimulator_R2021b/Command/Pilotage Horizontal/Pilotage Horizontal ==
  data: Flag input; command input; VehicleState input; Ac_rad input; Ac_out output; command_parameters parameter; SimuParameters parameter
function Ac_out = HorizontalControl(Flag,command,VehicleState,Ac_rad,command_parameters,SimuParameters)

persistent init memory;

horizontal_flag = GetFlagName(Flag.FlagHorizontal);

%% Load inputs
in.u_ms = VehicleState.nu.rAUV_WaterSpeed.Uwater_ms;
in.v_ms = VehicleState.nu.rAUV_WaterSpeed.Vwater_ms;
in.r_rads = VehicleState.nu.AngularSpeed.R_rads;
in.psi_rad = VehicleState.eta.EulerAngles.Psi_rad;
in.psic_rad = command;
in.delta_time_s = SimuParameters.sample_time_s;

%% Memory management
if isempty(init)
    init = false;
    memory = InitPilotHeading();
    Ac_rad = 0;
end
if init
    init = false;
    memory = InitPilotHeading();
end

%% Piloting
switch horizontal_flag
    case 'OpenLoop'
        Ac_rad = command;
        init = true;
        
    case 'Heading'
        horizontal_param = command_parameters.Horizontal.Heading;
        memory = UpdatePilotHeadingMemory(in, memory, horizontal_param);
        
        out = PilotHeading(in, memory, horizontal_param);
        Ac_rad = out.Ac;
end
Ac_out = Ac_rad;
end

function horizontal_flag = GetFlagName(flag)
% Get the horizontal_flag string depending on flag numeric input
horizontal_flag = '';

switch flag
    case 0
        horizontal_flag = 'OpenLoop';
    case 1
        horizontal_flag = 'Heading';
end
end

== matlab function MIR_AUVSimulator_R2021b/Command/Pilotage roulis/Pilotage roulis ==
  data: Flag input; command input; VehicleState input; Gc_rad input; Gc_out output; command_parameters parameter; SimuParameters parameter
function Gc_out = RollControl(Flag,command,VehicleState,Gc_rad,command_parameters,SimuParameters)

persistent init memory;

roll_flag = GetFlagName(Flag.FlagRoll);

%% Load inputs
in.u_ms = VehicleState.nu.rAUV_WaterSpeed.Uwater_ms;
in.p_rads = VehicleState.nu.AngularSpeed.P_rads;
in.phi_rad = VehicleState.eta.EulerAngles.Phi_rad;
in.phic_rad = command;
in.delta_time_s = SimuParameters.sample_time_s;

%% Memory management
if isempty(init)
    init = true;
    Gc_rad = 0;
    memory = InitPilotRoll();
end
if init
    init = false;
    memory = InitPilotRoll();
end

switch roll_flag
    case 'OpenLoop'
        Gc_rad = command;
        init = true;
        
    case 'Roll'
        roll_param = command_parameters.Roll;
        memory = UpdatePilotRollMemory(in, memory, roll_param);
        
        out = PilotRoll(in, memory, roll_param);
        Gc_rad = out.Gc;
end
Gc_out = Gc_rad;
end

function roll_flag = GetFlagName(flag)
% Get the roll_flag string depending on flag numeric input
roll_flag = '';

switch flag
    case 0
        roll_flag = 'OpenLoop';
    case 1
        roll_flag = 'Roll';
end
end

== matlab function MIR_AUVSimulator_R2021b/Vehicle Physics/Vehicle Dynamic/Add forces ==
  data: coriolis_forces input Bus: CoriolisForces; restoring_forces input Bus: RestoringForces; total_forces output Bus: TotalForces; hydrodynamic_forces input Bus: HydrodynamicForces; actuator_forces input Bus: ActuatorForces
function total_forces = fcn(coriolis_forces,restoring_forces,...
    hydrodynamic_forces, actuator_forces)

% Fields are : Fx_N, Fy_N, Fz_N an Mx_Nm, My_Nm, Mz_Nm

list_of_fields = fieldnames(coriolis_forces);
added_actuator_forces = AddActuatorsForces(actuator_forces);

for i=1:length(list_of_fields)
    fieldname = list_of_fields{i};
    
    total_forces.(fieldname) = added_actuator_forces.(fieldname) ...
        + coriolis_forces.(fieldname) + hydrodynamic_forces.(fieldname) ...
        + restoring_forces.(fieldname);
end
end

function output = AddActuatorsForces(actuator_forces)
% Fields are : HelmsForces and ThrusterForces
list_of_actuators = fieldnames(actuator_forces);

% Fields are : Fx_N, Fy_N, Fz_N an Mx_Nm, My_Nm, Mz_Nm
list_of_forces = fieldnames(actuator_forces.(list_of_actuators{1}));

% Init output
output = struct('Fx_N',0.0,'Fy_N',0.0,'Fz_N',0.0,'Mx_Nm',0.0,'My_Nm',0.0,'Mz_Nm',0.0);

for j=1:length(list_of_forces)
    force_name = list_of_forces{j};
    output.(force_name) = 0.0;
    for i=1:length(list_of_actuators)
        actuator = list_of_actuators{i};
        output.(force_name) = output.(force_name) + ...
            actuator_forces.(actuator).(force_name);
    end
end
end

== matlab function MIR_AUVSimulator_R2021b/Vehicle Physics/Modulo 2.Pi ==
  data: angle_in_rad input; angle_out_rad output
function angle_out_rad = Modulo2Pi(angle_in_rad)
% Heading is between 0° and 360° (we need to add a modulo)
angle_out_rad = mod(angle_in_rad,2*pi);

end

== matlab function MIR_AUVSimulator_R2021b/Vehicle Physics/Modulo 2.Pi1 ==
  data: angle_in_rad input; angle_out_rad output
function angle_out_rad = Modulo2Pi(angle_in_rad)
% Heading is between 0° and 360° (we need to add a modulo)
angle_out_rad = mod(angle_in_rad,2*pi);

end

== matlab function MIR_AUVSimulator_R2021b/Main thruster response to a setpoint ==
  data: Nc_sat_rpm input; struct_forces_out output Bus: ThrusterForces; veh_model parameter; WaterSpeed_ms input
function struct_forces_out = PropellerForces(Nc_sat_rpm,veh_model,WaterSpeed_ms)
% Be careful N°1: output need to be a struct (because bus) not an array
% Be careful n°2 : on units !
speed_ms = [WaterSpeed_ms.Uwater_ms;WaterSpeed_ms.Vwater_ms;WaterSpeed_ms.Wwater_ms];

%% Compute the force created by the thruster(=propeller)
thruster_forces = ComputePropellerForce(veh_model.Propeller,Nc_sat_rpm,speed_ms);
            
% Construct the struct output
struct_forces_out.Fx_N = thruster_forces(1);
struct_forces_out.Fy_N = thruster_forces(2);
struct_forces_out.Fz_N = thruster_forces(3);
struct_forces_out.Mx_Nm = thruster_forces(4);
struct_forces_out.My_Nm = thruster_forces(5);
struct_forces_out.Mz_Nm = thruster_forces(6);
end

== matlab function MIR_AUVSimulator_R2021b/Helms responses to bar angles/Repartitor ==
  data: Ac input; Gc input; B1c output; BARc input; veh_model parameter; B2c output; B3c output; B4c output; VehiculeState input
function [B1c,B2c,B3c,B4c] = Repartiteur(Ac,Gc,BARc,veh_model,VehiculeState)
% Transform virtual helms : BAR A and G to physical helms B1 B2 B3 and B4

inputs.Gc_rad = single(Gc);
inputs.BARc_rad = single(BARc);  
inputs.Ac_rad = single(Ac);
inputs.Phi_rad = VehiculeState.eta.EulerAngles.Phi_rad;

Out = ActuatorSetpoint(inputs, veh_model.XRearHelms.Bmax_rad);

B1c = double(Out.B1c_rad);
B2c = double(Out.B2c_rad);
B3c = double(Out.B3c_rad);
B4c = double(Out.B4c_rad);
end
